simulink model "vco_phase_noise"  (Simulink 7.4)
settings: Solver=ode45  StartTime=0.0  StopTime=.01  MaxStep=1/(4*50e6)  RelTol=1e-3
PreLoadFcn:
  | load f_inv;   % 1/f filter kernel
StopFcn:
  | plot_dbc_per_hz;
values from neighbouring files (symbols this model uses):
  Fs = OverSample*Freq(end)    [VCO_noise_profile_3.m]
undefined symbols (not defined in the file or in its folder): dBc, dfilt, Hz
libraries: dsparch4 x5, dspstat3 x3, simulink x2, dspbuff3 x2, dspsigops x2, dspspect3 x1, dspsnks4 x1, dspsrcs4 x1
settings Model: Creator=dbenson  LastModifiedBy=Dick
settings OptimizationCC: InlineInvariantSignals=on  InitFltsAndDblsToZero=on
settings DebuggingCC: SaveWithParameterizedLinksMsg=none  SignalResolutionControl=TryResolveAllWithWarning  MultiTaskDSMMsg=warning  MultiTaskCondExecSysMsg=none  StrictBusMsg=None
settings RTWCC: IncludeERTFirstTime=on
settings GRTTargetCC: TargetFcnLib=ansi_tfl_tmw.mat

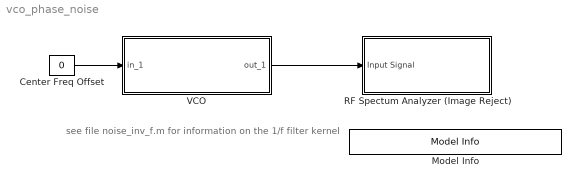
== system vco_phase_noise ==
  note: see file  noise_inv_f.m
      |   for information on the 1/f filter kernel
  Center Freq Offset : Constant  Value=0  VectorParams1D=off  OutDataType=sfix(16)  OutScaling=2^0
  Model Info : simulink/Model-Wide Utilities/Model Info  SystemSampleTime=-1  InitialBlockCM=None  BlockCM=None  Frame=on  DisplayStringWithTags=Copywrite 2005-2010 The MathWorks, Inc.  HorizontalTextAlignment=Center  LeftAlignmentValue=0.5  SourceBlockDiagram=vco_phase_noise  TagMaxNumber=20
  RF Spectum Analyzer (Image Reject) : Subsystem  Description=Spectrum Analyzer  mask{BW=4e6, Fc=49e6}
      mask prompts: BW "Bandwidth"; Fc "Center Freq"
      mask Display: fprintf('Spectrum Analyzer \n Fc=%7.2f MHz \n BW=%7.2f MHz',Fc/1e6,BW/1e6)
  VCO : Subsystem  mask{BW=2e6, Nrms=.01, Ph=0, Kc=1e6, Fc=49e6, Ac=1}
      mask prompts: BW "Single Sided Noise BW (Hz)"; Nrms "Phase Noise Level (rms rad)"; Ph "Initial Phase (rad)"; Kc "Input Sensitivity (Hz/Volt)"; Fc "Oscillation freq (Hz)"; Ac "Output amplitude (Volt)"
      mask init:
      | pi2=2*pi;
      mask Display: disp('VCO with \n 1/F phase noise')
  wires:
  VCO/1(out_1) -> RF Spectum Analyzer (Image Reject)/1(Input Signal)
  Center Freq Offset/1 -> VCO/1(in_1)

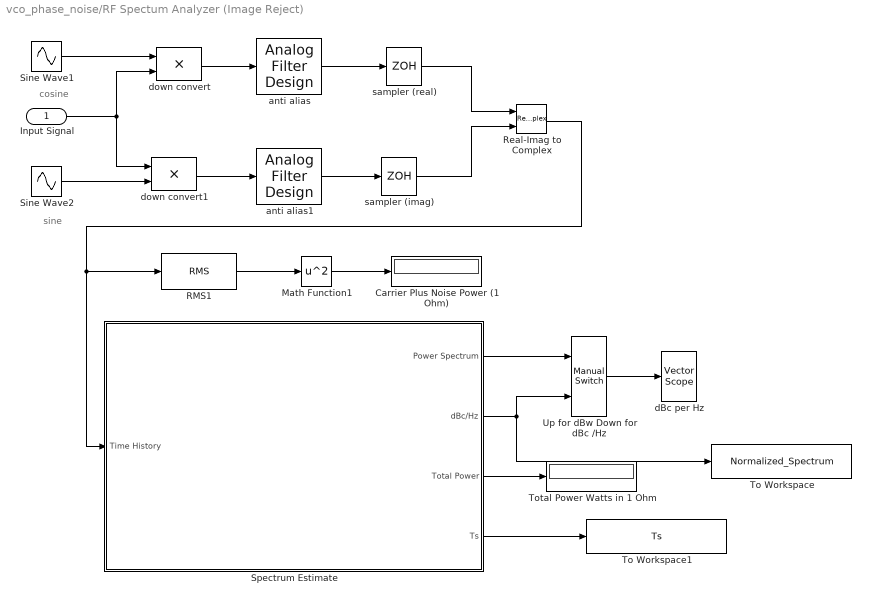
== system vco_phase_noise/RF Spectum Analyzer (Image Reject) ==
  note: cosine
  note: sine
  Input Signal : Inport  OutDataType=sfix(16)  OutScaling=2^0
  Carrier Plus Noise Power (1 Ohm) : Display
  Math Function1 : Math  Operator=square  OutDataType=sfix(16)  OutScaling=2^0  SaturateOnIntegerOverflow=on
  RMS1 : dspstat3/RMS  DialogController=dspDDGCreate  DialogControllerArgs=DataTag0  run=off  reset_popup=None  directionMode=Each column  dimension=1  treatSBRowAsCol=on
  Real-Imag to Complex : RealImagToComplex
  Sine Wave1 : Sin  Amplitude=1/7.2  Bias=0  Frequency=2*pi*(Fc)  Phase=-pi/2  Samples=10  SampleTime=0  Offset=0
  Sine Wave2 : Sin  Amplitude=1/7.2  Bias=0  Frequency=2*pi*(Fc)  Phase=0  Samples=10  SampleTime=0  Offset=0
  Spectrum Estimate : Subsystem  mask{Frame=1024, Navg=100}
      mask prompts: Frame "Frame Size"
      mask Display:
      | disp('Power Spectrum Estimate')
      | port_label('input',1,'y(t)');
      | port_label('output',1,'Power Spectrum')
      | port_label('output',2,'Scaled for dBc/Hz')
      | port_label('output',3','Total Power');
      | port_label('output',4','Ts');
  To Workspace : ToWorkspace  VariableName=Normalized_Spectrum  SampleTime=-1  SaveFormat=Array
      settings: MaxDataPoints=1
  To Workspace1 : ToWorkspace  VariableName=Ts  SampleTime=-1  SaveFormat=Array
      settings: MaxDataPoints=1
  Total Power Watts in 1 Ohm : Display
  Up for dBw Down for dBc /Hz : simulink/Signal Routing/Manual Switch  SystemSampleTime=-1  sw=0  action=0  varsize=off
  anti alias : dsparch4/Analog Filter Design  method=Elliptic  filttype=Lowpass  N=9  Wlo=BW*pi  Whi=80  Rp=1.2  Rs=100
  anti alias1 : dsparch4/Analog Filter Design  method=Elliptic  filttype=Lowpass  N=9  Wlo=BW*pi  Whi=80  Rp=1.2  Rs=100
  dBc per Hz : dspsnks4/Vector Scope  DialogController=dspdialog.VectorScope  DialogControllerArgs=DataTag4  ScopeProperties=on  Domain=Frequency  HorizSpan=1  DisplayProperties=off  AxisGrid=on  Memory=off  FrameNumber=on  AxisLegend=off  AxisZoom=off  OpenScopeAtSimStart=on  OpenScopeImmediately=off  FigPos=[26 68 560 252]  AxisProperties=off  XUnits=Hertz  XRange=[-Fs/2...Fs/2]  InheritXIncr=on  XIncr=1  XLabel=Time  XLimit=Auto  XMin=0  XMax=1  XStart=0  YUnits=dB  YLabel=dBc/Hz  LineProperties=off  XAxisParamsVer=6.9
      settings: YMin=-164.362362670898  YMax=2.17442076291263e-006
  down convert : Product  OutDataType=sfix(16)  OutScaling=2^0  SaturateOnIntegerOverflow=on  InputSameDT=on  OutDataTypeStr=Inherit: Same as first input
  down convert1 : Product  OutDataType=sfix(16)  OutScaling=2^0  SaturateOnIntegerOverflow=on  InputSameDT=on  OutDataTypeStr=Inherit: Same as first input
  sampler (imag) : ZeroOrderHold  SampleTime=1/(1.28*BW)
  sampler (real) : ZeroOrderHold  SampleTime=1/(1.28*BW)
  wires:
  Input Signal/1 -> down convert/2, down convert1/1
  down convert/1 -> anti alias/1
  anti alias/1 -> sampler (real)/1
  Sine Wave1/1 -> down convert/1
  Sine Wave2/1 -> down convert1/2
  anti alias1/1 -> sampler (imag)/1
  down convert1/1 -> anti alias1/1
  sampler (real)/1 -> Real-Imag to Complex/1
  sampler (imag)/1 -> Real-Imag to Complex/2
  Real-Imag to Complex/1 -> RMS1/1, Spectrum Estimate/1(Time History)
  Math Function1/1 -> Carrier Plus Noise Power (1 Ohm)/1
  Up for dBw Down for dBc /Hz/1 -> dBc per Hz/1
  Spectrum Estimate/3(Total Power) -> Total Power Watts in 1 Ohm/1
  Spectrum Estimate/2(dBc/Hz) -> Up for dBw Down for dBc /Hz/2, To Workspace/1
  Spectrum Estimate/1(Power Spectrum) -> Up for dBw Down for dBc /Hz/1
  RMS1/1 -> Math Function1/1
  Spectrum Estimate/4(Ts) -> To Workspace1/1

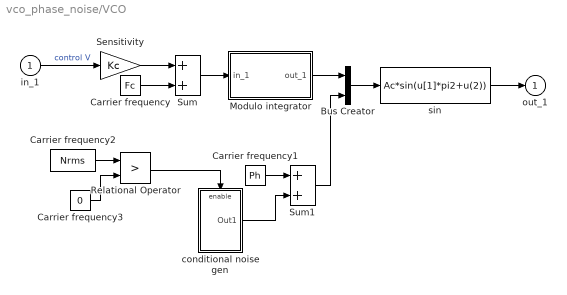
== system vco_phase_noise/VCO ==
  in_1 : Inport  OutDataType=sfix(16)  OutScaling=2^0
  Bus Creator : BusCreator  Inputs=2
  Carrier frequency : Constant  Value=Fc  OutDataType=sfix(16)  OutScaling=2^0
  Carrier frequency1 : Constant  Value=Ph  OutDataType=sfix(16)  OutScaling=2^0
  Carrier frequency2 : Constant  Value=Nrms  OutDataType=sfix(16)  OutScaling=2^0
  Carrier frequency3 : Constant  Value=0  OutDataType=sfix(16)  OutScaling=2^0
  Modulo integrator : Subsystem  mask(Modulo integrator){modu=1, init=0}
      mask prompts: modu "Modulo bound:"; init "Initial state:"
      mask help: When the absolute value of the state exceeds the modulo bound, the state is reset to be the remainder of the state divided by the modulo bound.
      mask Help: This block calculate the integration of the input signal. The absolute value of this integrator will not exceed the specified module bound. The state value is reset to be the remainder of the state divided by the modulo bound. This block can only be used for scale value calculation. This block is a continuous-time integration block.
      mask Display: disp('Modulo\nintegrator')
  Relational Operator : RelationalOperator  Operator=>  InputSameDT=on
  Sensitivity : Gain  Gain=Kc  ParameterDataType=sfix(16)  ParameterScaling=2^0  OutDataType=sfix(16)  OutScaling=2^0  SaturateOnIntegerOverflow=on  OutDataTypeStr=Inherit: Same as input  ParamDataTypeStr=Inherit: Same as input
  Sum : Sum  OutDataType=sfix(16)  OutScaling=2^0  SaturateOnIntegerOverflow=on  InputSameDT=on  OutDataTypeStr=Inherit: Same as first input
  Sum1 : Sum  OutDataType=sfix(16)  OutScaling=2^0  SaturateOnIntegerOverflow=on  InputSameDT=on  OutDataTypeStr=Inherit: Same as first input
  conditional noise gen : Subsystem  TreatAsAtomicUnit=on
  sin : Fcn  Expr=Ac*sin(u[1]*pi2+u(2))
  out_1 : Outport  OutDataType=sfix(16)  OutScaling=2^0
  wires:
  Modulo integrator/1(out_1) -> Bus Creator/1
  Bus Creator/1 -> sin/1
  Sum/1 -> Modulo integrator/1(in_1)
  sin/1 -> out_1/1
  Carrier frequency/1 -> Sum/2
  Sensitivity/1 -> Sum/1
  in_1/1 -> Sensitivity/1  "control V"
  Carrier frequency1/1 -> Sum1/1
  Sum1/1 -> Bus Creator/2
  conditional noise gen/1(Out1) -> Sum1/2
  Carrier frequency2/1 -> Relational Operator/1
  Relational Operator/1 -> conditional noise gen/Enable
  Carrier frequency3/1 -> Relational Operator/2

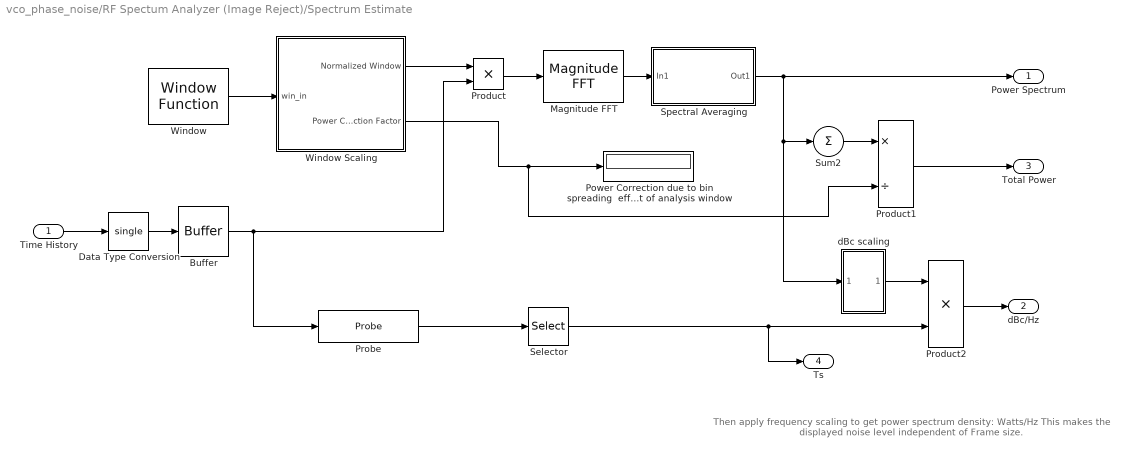
== system vco_phase_noise/RF Spectum Analyzer (Image Reject)/Spectrum Estimate ==
  note: Then apply frequency scaling to get power spectrum density: Watts/Hz
      | This makes the displayed noise level independent of Frame size.
  Time History : Inport  OutDataType=sfix(16)  OutScaling=2^0
  Buffer : dspbuff3/Buffer  N=Frame  V=0  ic=0
  Data Type Conversion : DataTypeConversion  OutDataTypeMode=single  OutDataType=sfix(16)  OutScaling=2^0  OutDataTypeStr=single
  Magnitude FFT : dspspect3/Magnitude FFT  SystemSampleTime=-1  mag_or_magsq=Magnitude squared  fftLenInherit=on  fftsize=fftsize
  "Power Correction due to bin spreading  effect of analysis window " : Display
  Probe : Probe  ProbeWidth=off  ProbeComplexSignal=off  ProbeWidthDataType=single  ProbeSampleTimeDataType=single
  Product : Product  OutDataType=sfix(16)  OutScaling=2^0  RndMeth=Zero
  Product1 : Product  Inputs=*/  OutDataType=sfix(16)  OutScaling=2^0  RndMeth=Zero
  Product2 : Product  Inputs=**  OutDataType=sfix(16)  OutScaling=2^0  RndMeth=Zero
  Selector : Selector  InputPortWidth=2  IndexOptions=Index vector (dialog)  Indices=[1]  OutputSizes=1
  Spectral Averaging : Subsystem  mask{Navg=100}
      mask Display: disp('Spectral Averaging')
  Sum2 : Sum  Inputs=+  OutDataType=sfix(16)  OutScaling=2^0
  Window : dspsigops/Window Function  DialogController=dspDDGCreate  DialogControllerArgs=DataTag2  winmode=Generate window  wintype=Hann  sampmode=Discrete  samptime=-1  N=Frame  Rs=60  beta=1  winsamp=Periodic  UserWindow=hamming  OptParams=off  UserParams={1.0}  dataType=single  isSigned=on  wordLen=16  udDataType=sfix(16)  fracBitsMode=Best precision  numFracBits=15  roundingMode=Floor  overflowMode=off  numSidelobes=4  sidelobeLevel=-30
      settings: additionalParams=on
  Window Scaling : Subsystem
  dBc scaling : Subsystem
  Power Spectrum : Outport  OutDataType=sfix(16)  OutScaling=2^0
  dBc/Hz : Outport  Port=2  OutDataType=sfix(16)  OutScaling=2^0
  Total Power : Outport  Port=3  OutDataType=sfix(16)  OutScaling=2^0
  Ts : Outport  Port=4  OutDataType=sfix(16)  OutScaling=2^0
  wires:
  Product/1 -> Magnitude FFT/1
  Magnitude FFT/1 -> Spectral Averaging/1(In1)
  Sum2/1 -> Product1/1
  Product1/1 -> Total Power/1
  Window/1 -> Window Scaling/1(win_in)
  Spectral Averaging/1(Out1) -> Power Spectrum/1, Sum2/1, dBc scaling/1(In1)
  Time History/1 -> Data Type Conversion/1
  dBc scaling/1(Out1) -> Product2/1
  Probe/1 -> Selector/1
  Product2/1 -> dBc/Hz/1
  Selector/1 -> Product2/2, Ts/1
  Data Type Conversion/1 -> Buffer/1
  Buffer/1 -> Probe/1, Product/2
  Window Scaling/1(Normalized Window) -> Product/1
  Window Scaling/2(Power Correction Factor) -> "Power Correction due to bin spreading  effect of analysis window "/1, Product1/2

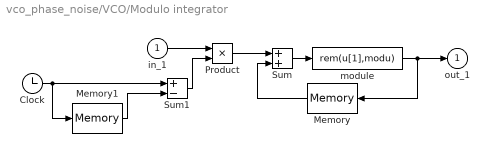
== system vco_phase_noise/VCO/Modulo integrator ==
  in_1 : Inport  OutDataType=sfix(16)  OutScaling=2^0
  Clock : Clock
      settings: Decimation=10
  Memory : Memory  X0=init
  Memory1 : Memory
  Product : Product  OutDataType=sfix(16)  OutScaling=2^0  SaturateOnIntegerOverflow=on  InputSameDT=on  OutDataTypeStr=Inherit: Same as first input
  Sum : Sum  OutDataType=sfix(16)  OutScaling=2^0  SaturateOnIntegerOverflow=on  InputSameDT=on  OutDataTypeStr=Inherit: Same as first input
  Sum1 : Sum  Inputs=+-  OutDataType=sfix(16)  OutScaling=2^0  SaturateOnIntegerOverflow=on  InputSameDT=on  OutDataTypeStr=Inherit: Same as first input
  module : Fcn  Expr=rem(u[1],modu)
  out_1 : Outport  OutDataType=sfix(16)  OutScaling=2^0
  wires:
  Memory1/1 -> Sum1/2
  Clock/1 -> Memory1/1, Sum1/1
  in_1/1 -> Product/1
  Sum1/1 -> Product/2
  Memory/1 -> Sum/2
  Product/1 -> Sum/1
  Sum/1 -> module/1
  module/1 -> out_1/1, Memory/1

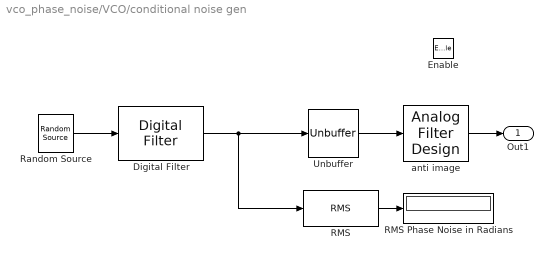
== system vco_phase_noise/VCO/conditional noise gen ==
  Enable : EnablePort
  Digital Filter : dsparch4/Digital Filter  DialogController=dspdialog.DigitalFilter  DialogControllerArgs=DataTag5  TypePopup=FIR (all zeros)  IIRFiltStruct=Direct form II transposed  AllPoleFiltStruct=Direct form  FIRFiltStruct=Direct form  CoeffSource=Specify via dialog  NumCoeffs=f_inv  DenCoeffs=[1 0.1]  BiQuadCoeffs=[1 0.3 0.4 1 0.1 0.2]  LatticeCoeffs=[0.2 0.4]  denIgnore=on  FiltPerSampPopup=One filter per frame  IC=0  ICnum=0  ICden=0  roundingMode=Floor  overflowMode=off  ScaleValues=1  scaleValueFracLength=14  stageInFracLength=15  stageOutFracLength=15  FilterSource=Specify via dialog  dfiltObjectName=dfilt.dffir([1 2 1])
  RMS : dspstat3/RMS  DialogController=dspDDGCreate  DialogControllerArgs=DataTag6  run=off  reset_popup=None  directionMode=Each column  dimension=1  treatSBRowAsCol=on
  RMS Phase Noise in Radians : Display
  Random Source : dspsrcs4/Random Source  SrcType=Gaussian  NormMethod=Ziggurat  CltLength=12  MinVal=0  MaxVal=1  MeanVal=0  VarVal=(Nrms)^2  RepMode=Not repeatable  rawSeed=1  IsInherit=off  SampMode=Discrete  SampTime=1/(2.56*BW)  SampFrame=512  DataType=Double  OutComplex=Real
  Unbuffer : dspbuff3/Unbuffer  ic=0
  anti image : dsparch4/Analog Filter Design  method=Elliptic  filttype=Lowpass  N=8  Wlo=BW*2*pi  Whi=80  Rp=2  Rs=100
  Out1 : Outport  OutDataType=sfix(16)  OutScaling=2^0
  wires:
  Random Source/1 -> Digital Filter/1
  Digital Filter/1 -> Unbuffer/1, RMS/1
  anti image/1 -> Out1/1
  Unbuffer/1 -> anti image/1
  RMS/1 -> RMS Phase Noise in Radians/1

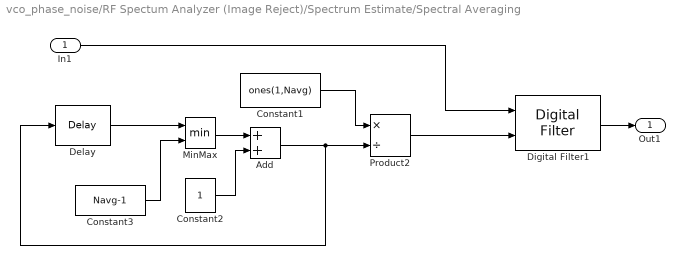
== system vco_phase_noise/RF Spectum Analyzer (Image Reject)/Spectrum Estimate/Spectral Averaging ==
  In1 : Inport  OutDataType=sfix(16)  OutScaling=2^0
  Add : Sum  OutDataType=sfix(16)  OutScaling=2^-10
  Constant1 : Constant  Value=ones(1,Navg)  OutDataTypeMode=single  OutDataType=sfix(16)  OutScaling=2^0  OutDataTypeStr=single
  Constant2 : Constant  OutDataTypeMode=single  OutDataType=sfix(16)  OutScaling=2^0  OutDataTypeStr=single  SampleTime=Frame/(1.28*BW)
  Constant3 : Constant  Value=Navg-1  OutDataTypeMode=single  OutDataType=sfix(16)  OutScaling=2^0  OutDataTypeStr=single  SampleTime=Frame/(1.28*BW)
  Delay : dspsigops/Delay  dly_unit=Samples  delay=1  ic_detail=off  dif_ic_for_ch=off  dif_ic_for_dly=off  ic=0  reset_popup=None
  Digital Filter1 : dsparch4/Digital Filter  DialogController=dspdialog.DigitalFilter  DialogControllerArgs=DataTag1  TypePopup=FIR (all zeros)  IIRFiltStruct=Direct form II transposed  AllPoleFiltStruct=Direct form  FIRFiltStruct=Direct form  CoeffSource=Input port(s)  NumCoeffs=[1 2]  DenCoeffs=[1 0.1]  BiQuadCoeffs=[1 0.3 0.4 1 0.1 0.2]  LatticeCoeffs=[0.2 0.4]  denIgnore=on  FiltPerSampPopup=One filter per frame  IC=0  ICnum=0  ICden=0  roundingMode=Floor  overflowMode=off  ScaleValues=1  scaleValueFracLength=14  stageInFracLength=15  stageOutFracLength=15  FilterSource=Input port(s)  dfiltObjectName=dfilt.dffir([1 2 1])
  MinMax : MinMax  Inputs=2  OutDataType=sfix(16)  OutScaling=2^0
  Product2 : Product  Inputs=*/  OutDataType=sfix(16)  OutScaling=2^0  RndMeth=Zero
  Out1 : Outport  OutDataType=sfix(16)  OutScaling=2^0
  wires:
  Add/1 -> Delay/1, Product2/2
  Constant2/1 -> Add/2
  Product2/1 -> Digital Filter1/2
  Delay/1 -> MinMax/1
  MinMax/1 -> Add/1
  Constant3/1 -> MinMax/2
  In1/1 -> Digital Filter1/1
  Digital Filter1/1 -> Out1/1
  Constant1/1 -> Product2/1

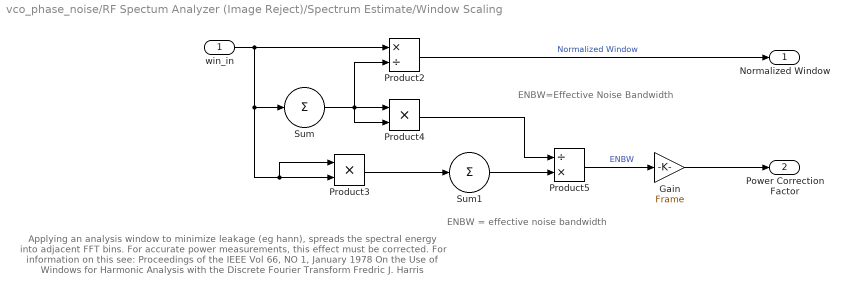
== system vco_phase_noise/RF Spectum Analyzer (Image Reject)/Spectrum Estimate/Window Scaling ==
  note: ENBW = effective noise bandwidth
  note: Applying an analysis window to minimize leakage (eg hann),
      | spreads the spectral energy into adjacent FFT bins.
      | For accurate power measurements, this effect must be corrected.
      | For information on this see:
      | Proceedings of the IEEE Vol 66, NO 1, January 1978
      | On the Use of Windows for Harmonic Analysis with the Discrete Fourier Transform
      | Fredric J. Harris
  note: ENBW=Effective Noise Bandwidth
  win_in : Inport  OutDataType=sfix(16)  OutScaling=2^0
  Gain : Gain  Gain=Frame  ParameterDataType=sfix(16)  ParameterScaling=2^0  OutDataType=sfix(16)  OutScaling=2^0
  Product2 : Product  Inputs=*/  OutDataType=sfix(16)  OutScaling=2^0  RndMeth=Zero
  Product3 : Product  OutDataType=sfix(16)  OutScaling=2^0  RndMeth=Zero
  Product4 : Product  OutDataType=sfix(16)  OutScaling=2^0  RndMeth=Zero
  Product5 : Product  Inputs=/*  OutDataType=sfix(16)  OutScaling=2^0  RndMeth=Zero
  Sum : Sum  Inputs=+  OutDataType=sfix(16)  OutScaling=2^0
  Sum1 : Sum  Inputs=+  OutDataType=sfix(16)  OutScaling=2^0
  Normalized Window : Outport  OutDataType=sfix(16)  OutScaling=2^0
  Power Correction Factor : Outport  Port=2  OutDataType=sfix(16)  OutScaling=2^0
  wires:
  Product2/1 -> Normalized Window/1  "Normalized Window"
  Product3/1 -> Sum1/1
  Product4/1 -> Product5/1
  Sum1/1 -> Product5/2
  Product5/1 -> Gain/1  "ENBW"
  win_in/1 -> Sum/1, Product3/1, Product3/2, Product2/1
  Sum/1 -> Product4/1, Product4/2, Product2/2
  Gain/1 -> Power Correction Factor/1

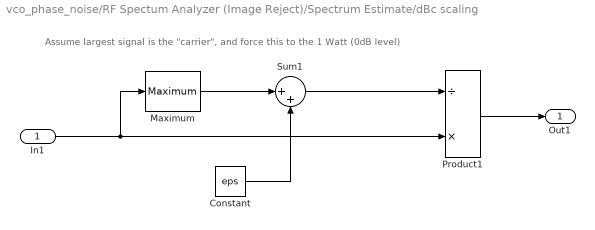
== system vco_phase_noise/RF Spectum Analyzer (Image Reject)/Spectrum Estimate/dBc scaling ==
  note: Assume largest signal is the "carrier", and force this to the 1 Watt (0dB level)
  In1 : Inport  OutDataType=sfix(16)  OutScaling=2^0
  Constant : Constant  Value=eps  OutDataType=sfix(16)  OutScaling=2^0
  Maximum : dspstat3/Maximum  DialogController=dspDDGCreate  DialogControllerArgs=DataTag3  fcn=Value  reset=None  indexBase=One  operateOver=Each column  Dimension=1  colComp=on  operation=maximum  roiEnable=off  roiType=Rectangles  roiPortion=Entire ROI  roiOutput=Individual statistics for each ROI  roiFlag=off  accumDataTypeStr=Inherit: Same as product output  accumLastDataTypeStr=Inherit: Same as product output  roundingMode=Floor  overflowMode=off
  Product1 : Product  Inputs=/*  OutDataType=sfix(16)  OutScaling=2^0  RndMeth=Zero
  Sum1 : Sum  Inputs=|++  OutDataType=sfix(16)  OutScaling=2^0
  Out1 : Outport  OutDataType=sfix(16)  OutScaling=2^0
  wires:
  In1/1 -> Maximum/1, Product1/2
  Product1/1 -> Out1/1
  Maximum/1 -> Sum1/1
  Sum1/1 -> Product1/1
  Constant/1 -> Sum1/2
